simulink model "cosim"  (R2013b)
settings: Solver=FixedStepDiscrete  SolverMode=SingleTasking  StartTime=0.0  StopTime=inf  FixedStep=0.01  RelTol=1e-3
undefined symbols (not defined in the file): A, N
libraries: xbsIndex_r4 x7, simulink x5, JTAGRuntimeCosim_r4 x1
settings Model: Creator=laca  LastModifiedBy=laca

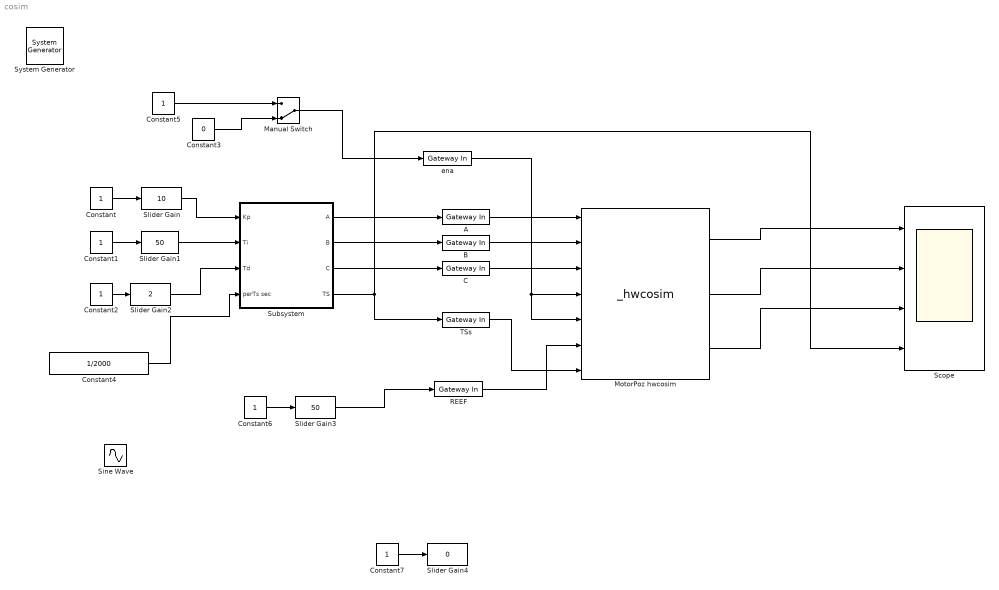
== system cosim ==
  " System Generator" : xbsIndex_r4/ System Generator  Tag=genX  xilinxfamily=spartan3e  part=xc3s500e  speed=-4  package=pq208  synthesis_tool=XST  clock_wrapper=Clock Enables  directory=./netlist  proj_type=Project Navigator  Synth_file=XST Defaults  Impl_file=ISE Defaults  testbench=off  simulink_period=1  sysclk_period=20  dcm_input_clock_period=10  incr_netlist=off  trim_vbits=Everywhere in SubSystem  dbl_ovrd=According to Block Masks  core_generation=According to Block Masks  run_coregen=off  deprecated_control=off  eval_field=0  block_type=sysgen
  A : xbsIndex_r4/Gateway In  gui_display_data_type=Fixed-point  arith_type=Unsigned  n_bits=16  bin_pt=0  preci_type=Single  exp_width=8  frac_width=24  quantization="Round  (unbiased: +/- Inf)"  overflow=Saturate  period=1  dbl_ovrd=off  timing_constraint=None  locs_specified=off  LOCs={}  UseAsADC=off  ADCChannel='1'  inherit_from_input=off  hdl_port=on  block_type=gatewayin
  B : xbsIndex_r4/Gateway In  gui_display_data_type=Fixed-point  arith_type=Unsigned  n_bits=16  bin_pt=0  preci_type=Single  exp_width=8  frac_width=24  quantization="Round  (unbiased: +/- Inf)"  overflow=Saturate  period=1  dbl_ovrd=off  timing_constraint=None  locs_specified=off  LOCs={}  UseAsADC=off  ADCChannel='1'  inherit_from_input=off  hdl_port=on  block_type=gatewayin
  C : xbsIndex_r4/Gateway In  gui_display_data_type=Fixed-point  arith_type=Unsigned  n_bits=16  bin_pt=0  preci_type=Single  exp_width=8  frac_width=24  quantization="Round  (unbiased: +/- Inf)"  overflow=Saturate  period=1  dbl_ovrd=off  timing_constraint=None  locs_specified=off  LOCs={}  UseAsADC=off  ADCChannel='1'  inherit_from_input=off  hdl_port=on  block_type=gatewayin
  Constant{,1..2,5..7} (6 alike) : Constant
  Constant3 : Constant  Value=0
  Constant4 : Constant  Value=1/2000
  Manual Switch : ManualSwitch  CurrentSetting=0
  MotorPoz hwcosim : JTAGRuntimeCosim_r4/_hwcosim  clkSrc=Free Running  hasCombinationalPath=on  bitfileName=C:\Users\laca\Desktop\iRoobo2014Ver3\Fpga\SPARTAN3E\Spartan3E6500SystemVer2\dcMOTORpositionPID\netlist\motorpoz_cw.bit  skipConfig=off  cable=Auto Detect  speed=N/A  cablePort=N/A  cableLocation=Local  shareCable=off  enable_codebug=on  design_xtable=|  engineDll=JTAGCosimEngine.dll  cableWaitTime=10  bscanPos=1  IRLengths=[6,8]  useWaitBox=1  hasBufgmux=on  Scheme=Cosim  useCmdProc=1  hasProc=0  useImpact=0  printLogFile=0  block_type=jtagcosim
      | {
      |   'clkWrapper' => 'motorpoz_cw',
      |   'clocksGcd' => undef,
      |   'device' => 'xc3s500e-4pq208',
      |   'ports' => {
      |     'aahj' => {
      |       'bd_port_index' => 0,
      |       'direction' => 'in',
      |       'icon_text' => 'Aahj',
      |       'period' => 1,
      |       'sim_pause_trigger' => false,
      |       'type' => 'UFix_16_0',
      |       'width' => 16,
      |     },
      |     'bb' => {
      |       'bd_port_index' => 1,
      |       'direction' => 'in',
      |       'icon_text' => 'Bb',
      |       'period' => 1,
      |       'sim_pause_trigger' => false,
      |       'type' => 'UFix_16_0',
      |       'width' => 16,
      |     },
      |     'cc' => {
      |       'bd_port_index' => 2,
      |       'direction' => 'in',
      |       'icon_text' => 'Cc',
      |       'period' => 1,
      |       'sim_pause_trigger' => false,
      |       'type' => 'UFix_16_0',
      |       'width' => 16,
      |     },
      |     'counterval' => {
      |       'bd_port_index' => 0,
      |       'direction' => 'out',
      |       'icon_text' => 'counterval',
      |       'period' => 1,
      |       'sim_pause_trigger' => false,
      |       'type' => 'Fix_16_0',
      |       'width' => 16,
      |     },
      |     'direct_inp' => {
      |       'bd_port_index' => 3,
      |       'direction' => 'in',
      |       'icon_text' => 'direct inp',
      |       'period' => 1,
      |       'sim_pause_trigger' => false,
      |       'type' => 'Bool',
      |       'width' => 1,
      |     },
      |     'e' => {
      |       'bd_port_index' => 1,
      |       'direction' => 'out',
      |       'icon_text' => 'e',
      |       'period' => 1,
      |       'sim_pause_trigger' => false,
      |       'type' => 'Fix_17_0',
      |       'width' => 17,
      |     },
      |     'enapwm' => {
      |       'bd_port_index' => 4,
      |       'direction' => 'in',
      |       'icon_text' => 'enapwm',
      |       'period' => 1,
      |       'sim_pause_trigger' => false,
      |       'type' => 'Bool',
      |       'width' => 1,
      |     },
      |     'recerencia' => {
      |       'bd_port_index' => 5,
      |       'direction' => 'in',
      |       'icon_text' => 'recerencia',
      |       'period' => 1,
      |       'sim_pause_trigger' => false,
      |       'type' => 'Fix_16_0',
      |       'width' => 16,
      |     },
      |     'ts' => {
      |       'bd_port_index' => 6,
      |       'direction' => 'in',
      |       'icon_text' => 'TS',
      |       'period' => 1,
      |       'sim_pause_trigger' => false,
      |       'type' => 'UFix_32_0',
      |       'width' => 32,
      |     },
      |     'u' => {
      |       'bd_port_index' => 2,
      |       'direction' => 'out',
      |       'icon_text' => 'u',
      |       'period' => 1,
      |       'sim_pause_trigger' => false,
      |       'type' => 'Fix_17_0',
      |       'width' => 17,
      |     },
      |   },
      |   'shared_memories' => {},
      | }
  REEF : xbsIndex_r4/Gateway In  gui_display_data_type=Fixed-point  arith_type="Signed  (2's comp)"  n_bits=16  bin_pt=0  preci_type=Single  exp_width=8  frac_width=24  quantization="Round  (unbiased: +/- Inf)"  overflow=Saturate  period=1  dbl_ovrd=off  timing_constraint=None  locs_specified=off  LOCs={}  UseAsADC=off  ADCChannel='1'  inherit_from_input=off  hdl_port=on  block_type=gatewayin
  Scope : Scope  NumInputPorts=4
      settings: YMin=-88.2~-2.1~-27480~237500  YMax=-79.8~-1.9~-27437.5~262500  SaveName=ScopeData2
  Sine Wave : Sin  Amplitude=50  Frequency=0.001  SampleTime=1
  Slider Gain : simulink/Math Operations/Slider Gain  low=0  gain=10  high=65000
  Slider Gain1 : simulink/Math Operations/Slider Gain  low=0  gain=50  high=65000
  Slider Gain2 : simulink/Math Operations/Slider Gain  low=0  gain=2  high=5000
  Slider Gain3 : simulink/Math Operations/Slider Gain  low=-180  gain=50  high=180
  Slider Gain4 : simulink/Math Operations/Slider Gain  low=0  gain=0  high=65530
  Subsystem : Subsystem
  TSs : xbsIndex_r4/Gateway In  gui_display_data_type=Fixed-point  arith_type=Unsigned  n_bits=32  bin_pt=0  preci_type=Single  exp_width=8  frac_width=24  quantization="Round  (unbiased: +/- Inf)"  overflow=Saturate  period=1  dbl_ovrd=off  timing_constraint=None  locs_specified=off  LOCs={}  UseAsADC=off  ADCChannel='1'  inherit_from_input=off  hdl_port=on  block_type=gatewayin
  ena : xbsIndex_r4/Gateway In  gui_display_data_type=Boolean  arith_type=Boolean  n_bits=16  bin_pt=0  preci_type=Single  exp_width=8  frac_width=24  quantization="Round  (unbiased: +/- Inf)"  overflow=Saturate  period=1  dbl_ovrd=off  timing_constraint=None  locs_specified=off  LOCs={}  UseAsADC=off  ADCChannel='1'  inherit_from_input=off  hdl_port=on  block_type=gatewayin
  wires:
  MotorPoz hwcosim/2 -> Scope/2
  MotorPoz hwcosim/3 -> Scope/3
  Constant/1 -> Slider Gain/1
  Constant1/1 -> Slider Gain1/1
  Constant2/1 -> Slider Gain2/1
  A/1 -> MotorPoz hwcosim/1
  C/1 -> MotorPoz hwcosim/3
  B/1 -> MotorPoz hwcosim/2
  Subsystem/1(A) -> A/1
  Subsystem/2(B) -> B/1
  Subsystem/3(C) -> C/1
  Subsystem/4(TS) -> TSs/1, Scope/4
  Slider Gain/1 -> Subsystem/1(Kp)
  Slider Gain1/1 -> Subsystem/2(Ti)
  Slider Gain2/1 -> Subsystem/3(Td)
  Constant4/1 -> Subsystem/4(perTs sec)
  MotorPoz hwcosim/1 -> Scope/1
  Manual Switch/1 -> ena/1
  Constant5/1 -> Manual Switch/1
  Constant3/1 -> Manual Switch/2
  Constant6/1 -> Slider Gain3/1
  Slider Gain3/1 -> REEF/1
  TSs/1 -> MotorPoz hwcosim/7
  REEF/1 -> MotorPoz hwcosim/6
  Constant7/1 -> Slider Gain4/1
  ena/1 -> MotorPoz hwcosim/4, MotorPoz hwcosim/5

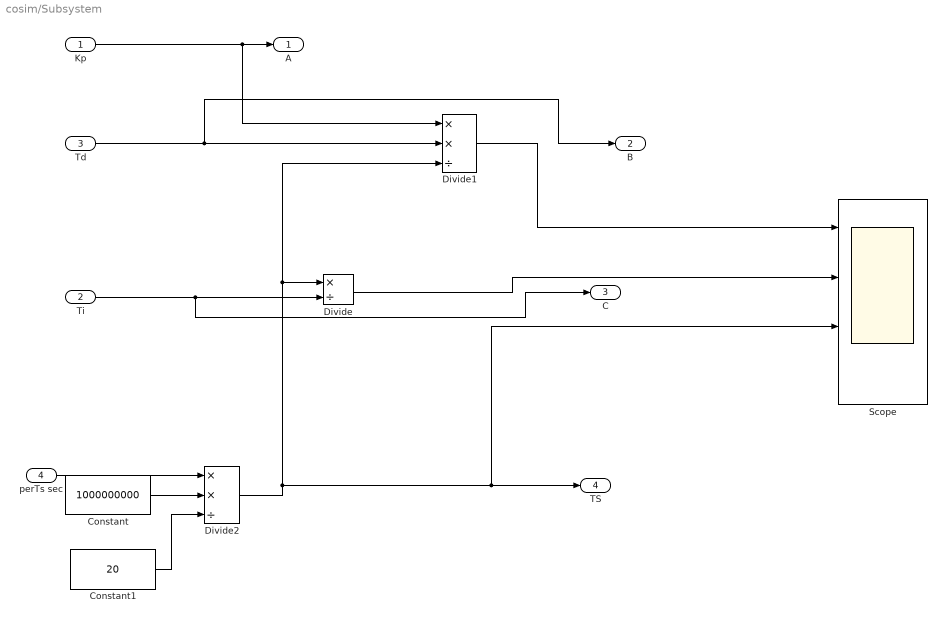
== system cosim/Subsystem ==
  Kp : Inport
  Ti : Inport  Port=2
  Td : Inport  Port=3
  perTs sec : Inport  Port=4
  Constant : Constant  Value=1000000000
  Constant1 : Constant  Value=20
  Divide : Product  Inputs=*/
  Divide1 : Product  Inputs=**/
  Divide2 : Product  Inputs=**/
  Scope : Scope  NumInputPorts=4
      settings: YMin=1.3659~1.7179~2375~237.5  YMax=1.50968~1.89874~2625~262.5
  A : Outport
  B : Outport  Port=2
  C : Outport  Port=3
  TS : Outport  Port=4
  wires:
  Kp/1 -> Divide1/1, A/1
  Divide2/1 -> Scope/3, TS/1, Divide1/3, Divide/1
  Ti/1 -> C/1, Divide/2
  Divide/1 -> Scope/2
  Td/1 -> B/1, Divide1/2
  Divide1/1 -> Scope/1
  perTs sec/1 -> Divide2/1
  Constant/1 -> Divide2/2
  Constant1/1 -> Divide2/3
